simulink model "PMS_Motor_level3eZDSPF2812"  (Simulink 6.5)
settings: Solver=FixedStepDiscrete  StartTime=0.0  StopTime=0.3  RelTol=1e-3
libraries: c28xdmclib x6, simulink x5, tiiqmathlib x4, c281xdspchiplib x3, c2000tgtpreflib x1
CloseFcn:
  | rtwprivate ssgencode ModelCloseRequest Simple_DC_Motor
settings Model: Creator=JacobF  LastModifiedBy=JacobF  ProdHWDeviceType=TI C2000
settings DataIOCC: SaveOutput=off  SaveTime=off  SignalLoggingName=DataLog
settings OptimizationCC: OptimizeModelRefInitCode=on  LifeSpan=1
settings DebuggingCC: ReadBeforeWriteMsg=DisableAll  MultiTaskDSMMsg=warning  MultiTaskCondExecSysMsg=none  ParameterPrecisionLossMsg=none  StrictBusMsg=ErrorLevel1
settings HardwareCC: ProdBitPerChar=16  ProdBitPerInt=16  ProdIntDivRoundTo=Zero  ProdEndianess=LittleEndian  ProdWordSize=16  ProdHWDeviceType=TI C2000  TargetHWDeviceType=32-bit Generic
settings RTWCC: SystemTargetFile=ti_c2000_ert.tlc  GenCodeOnly=on  TemplateMakefile=ti_c2000_ert.tmf  Description=Embedded Target for TI C2000 DSP (ERT)  GenerateReport=on  ProcessScript=ti_c2000_ert_make_rtw_hook  IncludeHyperlinkInReport=on  LaunchReport=on
settings CodeAppCC: IgnoreCustomStorageClasses=off
settings STFCustomTargetCC: TargetFcnLib=ansi_tfl_tmw.mat  GenFloatMathFcnCalls=ANSI_C  ModelReferenceCompliant=off  CombineOutputUpdateFcns=on  ERTCustomFileBanners=on  SystemTargetFile=ti_c2000_ert.tlc
settings ERTTargetCC: TargetFcnLib=ansi_tfl_tmw.mat  GenFloatMathFcnCalls=ANSI_C  ModelReferenceCompliant=off  SupportContinuousTime=on  SupportNonInlinedSFcns=on  InlinedParameterPlacement=NonHierarchical  ERTCustomFileTemplate=example_file_process.tlc

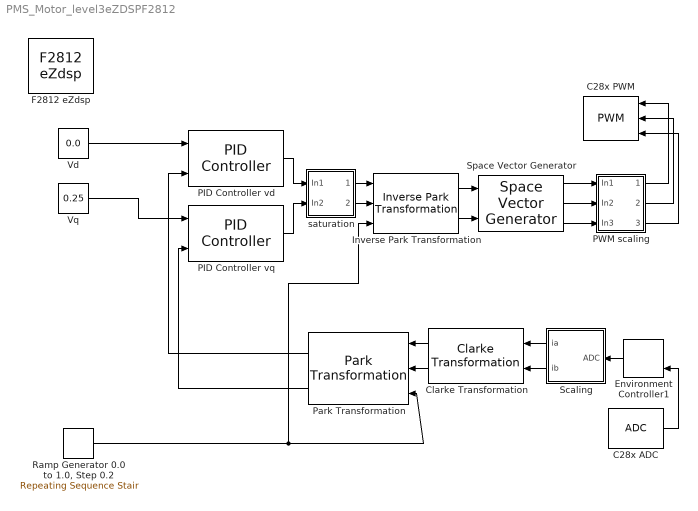
== system PMS_Motor_level3eZDSPF2812 ==
  C28x ADC : c281xdspchiplib/ADC  useModule=A  useMode=Sequential  sourceSOC=Software  Ts=-1  dType=uint16  postInterrupt=off  numConversionsSingle=3  numConversionsDouble=1  conv0=ADCINB0  conv1=ADCINB1  conv2=ADCINB2  conv3=ADCINB3  conv4=ADCINA4  conv5=ADCINA5  conv6=ADCINB6  conv7=ADCINA7  conv8=ADCINB0  conv9=ADCINB1  conv10=ADCINB2  conv11=ADCINB3  conv12=ADCINB4  conv13=ADCINB5  conv14=ADCINB6  conv15=ADCINB7  convAB0=ADCINA0 and ADCINB0  convAB1=ADCINA1 and ADCINB1  convAB2=ADCINA5 and ADCINB5  convAB3=ADCINA1 and ADCINB1  convAB4=ADCINA1 and ADCINB1  convAB5=ADCINA1 and ADCINB1  convAB6=ADCINA1 and ADCINB1  convAB7=ADCINA1 and ADCINB1  convA0=ADCINA0  convA1=ADCINA1  convA2=ADCINA7  convA3=ADCINA3  convA4=ADCINA4  convA5=ADCINA5  convA6=ADCINA6  convA7=ADCINA7  convB0=ADCINB0  convB1=ADCINB1  convB2=ADCINB2  convB3=ADCINB3  convB4=ADCINB4  convB5=ADCINB5  convB6=ADCINB6  convB7=ADCINB7  c28xmultiPort=off
  C28x PWM : c281xdspchiplib/PWM  Orientation=left  useModule=A  timerSource=Specify via dialog  timerPeriod=(2^12)+1  waveformType=Symmetric  periodUnits=Clock cycles  unit1Status=on  unit1Source=Input port  unit1Value=4096  unit2Status=on  unit2Source=Input port  unit2Value=4096  unit3Status=on  unit3Source=Input port  unit3Value=4096  dutyCycleUnits=Clock cycles  logicSource=Specify via dialog  unit1_1Logic=Active high  unit1_2Logic=Active low  unit2_1Logic=Active high  unit2_2Logic=Active low  unit3_1Logic=Active high  unit3_2Logic=Active low  enableDeadband1=on  enableDeadband2=on  enableDeadband3=on  deadbandPrescaler=8  deadbandPeriodSource=Specify via dialog  deadbandPeriod=15  adcstartEvent=None
  Clarke Transformation : c28xdmclib/Clarke Transformation  Orientation=left
  Environment Controller1 : simulink/Signal Routing/Environment Controller  Orientation=left  SystemSampleTime=-1
  F2812 eZdsp : c2000tgtpreflib/F2812 eZdsp  Tag=C2000 TARGET PREFERENCES BLOCK  SystemSampleTime=-1
  Inverse Park Transformation : c28xdmclib/Inverse Park Transformation
  PID Controller vd : c28xdmclib/PID Controller  proportionalGain=0.2  integralGain=0.002  correctionGain=0.002  derivativeGain=0  minOutput=-1  maxOutput=1
  PID Controller vq : c28xdmclib/PID Controller  proportionalGain=0.2  integralGain=0.002  correctionGain=0.002  derivativeGain=0  minOutput=-1  maxOutput=1
  PWM scaling : Subsystem
  Park Transformation : c28xdmclib/Park Transformation  Orientation=left
  "Ramp Generator 0.0 to 1.0, Step 0.2" : simulink/Sources/Repeating Sequence Stair  SystemSampleTime=-1  OutValues=[0.0:0.0005:1.0]  tsamp=0.00005  OutputDataTypeScalingMode=Specify via dialog  OutDataType=sfix(32)  ConRadixGroup=Use Specified Scaling  OutScaling=2^-17
  Scaling : Subsystem  Orientation=left
  Space Vector Generator : c28xdmclib/Space Vector Generator
  Vd : Constant  Value=0.0  OutDataTypeMode=Specify via dialog  OutDataType=sfix(32)  ConRadixGroup=Use specified scaling  OutScaling=2^-17  SampleTime=inf  FramePeriod=inf
  Vq : Constant  Value=0.25  OutDataTypeMode=Specify via dialog  OutDataType=sfix(32)  ConRadixGroup=Use specified scaling  OutScaling=2^-17  SampleTime=inf  FramePeriod=inf
  saturation : Subsystem
  wires:
  Inverse Park Transformation/1 -> Space Vector Generator/1
  Inverse Park Transformation/2 -> Space Vector Generator/2
  Space Vector Generator/1 -> PWM scaling/1(In1)
  Space Vector Generator/2 -> PWM scaling/2(In2)
  Space Vector Generator/3 -> PWM scaling/3(In3)
  PWM scaling/1(Out1) -> C28x PWM/1
  PWM scaling/2(Out2) -> C28x PWM/2
  PWM scaling/3(Out3) -> C28x PWM/3
  Environment Controller1/1 -> Scaling/1(ADC)
  C28x ADC/1 -> Environment Controller1/2
  Scaling/1(ia) -> Clarke Transformation/1
  Scaling/2(ib) -> Clarke Transformation/2
  Clarke Transformation/1 -> Park Transformation/1
  Clarke Transformation/2 -> Park Transformation/2
  PID Controller vd/1 -> saturation/1(In1)
  PID Controller vq/1 -> saturation/2(In2)
  Vd/1 -> PID Controller vd/1
  Park Transformation/1 -> PID Controller vd/2
  Park Transformation/2 -> PID Controller vq/2
  saturation/1(Out1) -> Inverse Park Transformation/1
  saturation/2(Out2) -> Inverse Park Transformation/2
  Vq/1 -> PID Controller vq/1
  "Ramp Generator 0.0 to 1.0, Step 0.2"/1 -> Inverse Park Transformation/3, Park Transformation/3

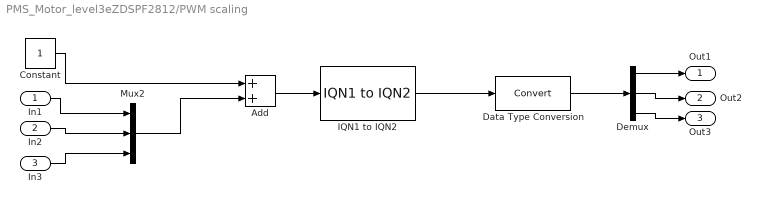
== system PMS_Motor_level3eZDSPF2812/PWM scaling ==
  In1 : Inport
  In2 : Inport  Port=2
  In3 : Inport  Port=3
  Add : Sum  OutScaling=2^-10
  Constant : Constant  Value=1  OutDataTypeMode=Specify via dialog  OutDataType=sfix(32)  ConRadixGroup=Use specified scaling  OutScaling=2^-17  SampleTime=inf  FramePeriod=inf
  Data Type Conversion : DataTypeConversion  OutDataTypeMode=uint16  ConvertRealWorld=Stored Integer (SI)
  Demux : Demux  Outputs=3
  IQN1 to IQN2 : tiiqmathlib/IQN1 to IQN2  New_Q=11
  Mux2 : Mux  Inputs=3
  Out1 : Outport
  Out2 : Outport  Port=2
  Out3 : Outport  Port=3
  wires:
  In1/1 -> Mux2/1
  Add/1 -> IQN1 to IQN2/1
  Constant/1 -> Add/1
  IQN1 to IQN2/1 -> Data Type Conversion/1
  In3/1 -> Mux2/3
  In2/1 -> Mux2/2
  Mux2/1 -> Add/2
  Data Type Conversion/1 -> Demux/1
  Demux/3 -> Out3/1
  Demux/2 -> Out2/1
  Demux/1 -> Out1/1

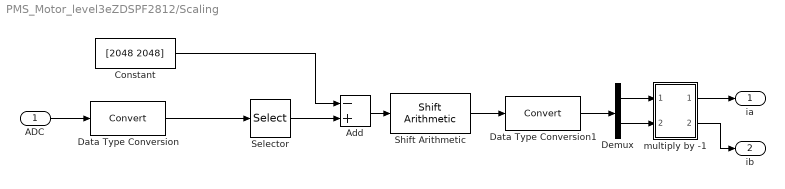
== system PMS_Motor_level3eZDSPF2812/Scaling ==
  ADC : Inport
  Add : Sum  Inputs=-+  OutScaling=2^-10
  Constant : Constant  Value=[2048 2048]  OutDataTypeMode=int32  OutDataType=sfix(32)  ConRadixGroup=Use specified scaling  OutScaling=2^-12  SampleTime=inf  FramePeriod=inf
  Data Type Conversion : DataTypeConversion  OutDataTypeMode=int32  OutDataType=sfix(32)  OutScaling=2^-12  ConvertRealWorld=Stored Integer (SI)
  Data Type Conversion1 : DataTypeConversion  OutDataTypeMode=Specify via dialog  OutDataType=sfix(32)  OutScaling=2^-17  ConvertRealWorld=Stored Integer (SI)
  Demux : Demux  Outputs=2
  Selector : Selector  InputType=Vector  ElementSrc=Internal  Elements=[1 2]  RowSrc=Internal  Rows=1  ColumnSrc=Internal  Columns=1  InputPortWidth=3  IndexIsStartValue=off
  Shift Arithmetic : simulink/Logic and Bit Operations/Shift Arithmetic  SystemSampleTime=-1  nBitShiftRight=-6  nBinPtShiftRight=0
  multiply by -1 : Subsystem
  ia : Outport
  ib : Outport  Port=2
  wires:
  ADC/1 -> Data Type Conversion/1
  multiply by -1/2(Out2) -> ib/1
  multiply by -1/1(Out1) -> ia/1
  Demux/2 -> multiply by -1/2(In2)
  Demux/1 -> multiply by -1/1(In1)
  Data Type Conversion1/1 -> Demux/1
  Shift Arithmetic/1 -> Data Type Conversion1/1
  Add/1 -> Shift Arithmetic/1
  Selector/1 -> Add/2
  Constant/1 -> Add/1
  Data Type Conversion/1 -> Selector/1

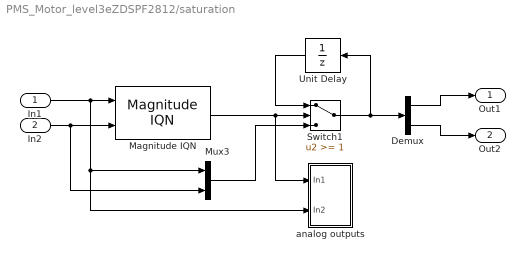
== system PMS_Motor_level3eZDSPF2812/saturation ==
  In1 : Inport
  In2 : Inport  Port=2
  Demux : Demux  Outputs=2
  Magnitude IQN : tiiqmathlib/Magnitude IQN
  Mux3 : Mux  Inputs=2
  Switch1 : Switch  Threshold=1
  Unit Delay : UnitDelay  Orientation=left  X0=[0 0]  SampleTime=-1
  analog outputs : Subsystem
  Out1 : Outport
  Out2 : Outport  Port=2
  wires:
  Magnitude IQN/1 -> Switch1/2, analog outputs/1(In1)
  In1/1 -> Magnitude IQN/1, Mux3/1, analog outputs/2(In2)
  In2/1 -> Magnitude IQN/2, Mux3/2
  Mux3/1 -> Switch1/3
  Switch1/1 -> Unit Delay/1, Demux/1
  Unit Delay/1 -> Switch1/1
  Demux/1 -> Out1/1
  Demux/2 -> Out2/1

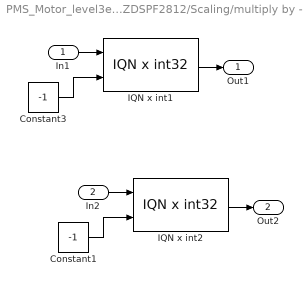
== system PMS_Motor_level3eZDSPF2812/Scaling/multiply by -1 ==
  In1 : Inport
  In2 : Inport  Port=2
  Constant1 : Constant  Value=-1  OutDataTypeMode=int32  OutDataType=sfix(32)  ConRadixGroup=Use specified scaling  OutScaling=2^-17  SampleTime=inf  FramePeriod=inf
  Constant3 : Constant  Value=-1  OutDataTypeMode=int32  OutDataType=sfix(32)  ConRadixGroup=Use specified scaling  OutScaling=2^-17  SampleTime=inf  FramePeriod=inf
  IQN x int1 : tiiqmathlib/IQN x int32
  IQN x int2 : tiiqmathlib/IQN x int32
  Out1 : Outport
  Out2 : Outport  Port=2
  wires:
  IQN x int2/1 -> Out2/1
  In2/1 -> IQN x int2/1
  Constant1/1 -> IQN x int2/2
  IQN x int1/1 -> Out1/1
  In1/1 -> IQN x int1/1
  Constant3/1 -> IQN x int1/2

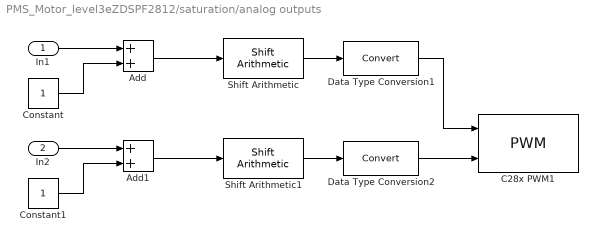
== system PMS_Motor_level3eZDSPF2812/saturation/analog outputs ==
  In1 : Inport
  In2 : Inport  Port=2
  Add : Sum  OutScaling=2^-10
  Add1 : Sum  OutScaling=2^-10
  C28x PWM1 : c281xdspchiplib/PWM  useModule=B  timerSource=Specify via dialog  timerPeriod=37500  waveformType=Symmetric  periodUnits=Clock cycles  unit1Status=on  unit1Source=Input port  unit1Value=18500  unit2Status=on  unit2Source=Input port  unit2Value=18500  unit3Status=off  unit3Source=Input port  unit3Value=18500  dutyCycleUnits=Clock cycles  logicSource=Specify via dialog  unit1_1Logic=Active high  unit1_2Logic=Active low  unit2_1Logic=Active high  unit2_2Logic=Active low  unit3_1Logic=Active high  unit3_2Logic=Active low  enableDeadband1=on  enableDeadband2=on  enableDeadband3=on  deadbandPrescaler=8  deadbandPeriodSource=Specify via dialog  deadbandPeriod=15  adcstartEvent=None
  Constant : Constant  Value=1  OutDataTypeMode=Specify via dialog  OutDataType=sfix(32)  ConRadixGroup=Use specified scaling  OutScaling=2^-17  SampleTime=inf  FramePeriod=inf
  Constant1 : Constant  Value=1  OutDataTypeMode=Specify via dialog  OutDataType=sfix(32)  ConRadixGroup=Use specified scaling  OutScaling=2^-17  SampleTime=inf  FramePeriod=inf
  Data Type Conversion1 : DataTypeConversion  OutDataTypeMode=uint16  OutDataType=sfix(32)  OutScaling=2^-17  ConvertRealWorld=Stored Integer (SI)
  Data Type Conversion2 : DataTypeConversion  OutDataTypeMode=uint16  OutDataType=sfix(32)  OutScaling=2^-17  ConvertRealWorld=Stored Integer (SI)
  Shift Arithmetic : simulink/Logic and Bit Operations/Shift Arithmetic  SystemSampleTime=-1  nBitShiftRight=3  nBinPtShiftRight=0
  Shift Arithmetic1 : simulink/Logic and Bit Operations/Shift Arithmetic  SystemSampleTime=-1  nBitShiftRight=3  nBinPtShiftRight=0
  wires:
  In1/1 -> Add/1
  Constant/1 -> Add/2
  Add/1 -> Shift Arithmetic/1
  Shift Arithmetic/1 -> Data Type Conversion1/1
  Data Type Conversion1/1 -> C28x PWM1/1
  In2/1 -> Add1/1
  Constant1/1 -> Add1/2
  Add1/1 -> Shift Arithmetic1/1
  Shift Arithmetic1/1 -> Data Type Conversion2/1
  Data Type Conversion2/1 -> C28x PWM1/2
